simulink model "Velocity_PI"  (R2024b)
settings: Solver=VariableStepAuto  StartTime=0.0  StopTime=30  RelTol=1e-3
settings Model: Creator=simon  LastModifiedBy=simon

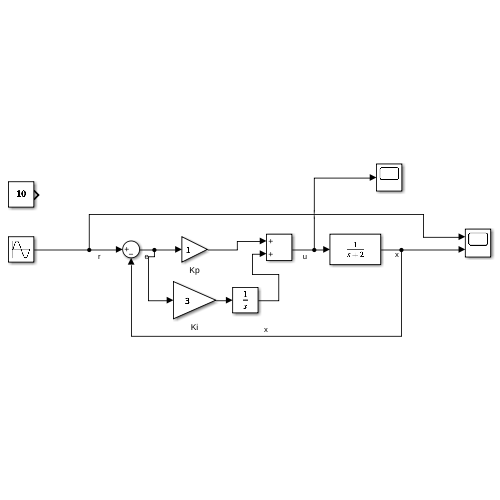
[thumbnail: Simulink's stored preview of the top-level diagram]
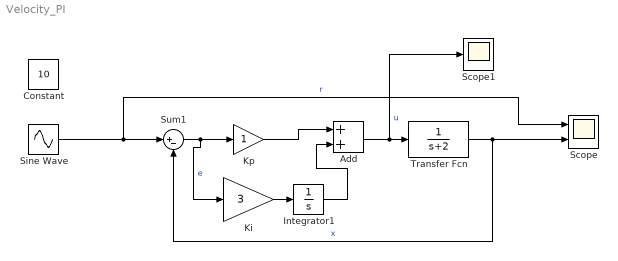
== system Velocity_PI ==
  Add : Sum
  Constant : Constant  Value=10
  Integrator1 : Integrator
  Ki : Gain  Gain=3
  Kp : Gain
  Scope : Scope  NumInputPorts=2
  Scope1 : Scope
  Sine Wave : Sin  Amplitude=3  SampleTime=0
  Sum1 : Sum  Inputs=|+-
  Transfer Fcn : TransferFcn  Denominator=[1 2]
  wires:
  Sum1/1 -> Ki/1, Kp/1  "e"
  Transfer Fcn/1 -> Scope/2, Sum1/2  "x"
  Sine Wave/1 -> Scope/1, Sum1/1  "r"
  Kp/1 -> Add/1
  Integrator1/1 -> Add/2
  Add/1 -> Scope1/1, Transfer Fcn/1  "u"
  Ki/1 -> Integrator1/1
